simulink model "M4B11_modified_AGC_PI"  (R2025a)
settings: Solver=VariableStepAuto  StartTime=0.0  StopTime=100  RelTol=1e-3
InitFcn:
  | clear;
  | load('parameterinit.mat');
  | set_param('M4B11_modified_AGC_PI/Python2Sim','value','[0 0 0 0 0 0 0 0]');
  | acom=100;
  | bcom=50;
  | lam=100;
values from neighbouring files (symbols this model uses):
  ACgirdinit =     [datainit.mat]    (also in parameterinit.mat)
  AVm0 = [11.3576294988 11.3576294988]    [datainit.mat]    (also in parameterinit.mat)
  commun = [1 1 1 0]    [datainit.mat]    (also in initAll.m = [1,1,1,0]; parameterinit.mat)
  DataDelay = [0  0; 0  0; 0  0; 0  0]    [datainit.mat]    (also in initAll.m = 0.0*DataDelay; parameterinit.mat)
  ESinit =     [datainit.mat]    (also in parameterinit.mat)
  fB = 50    [datainit.mat]    (also in initAll.m; parameterinit.mat)
  Geninit =     [datainit.mat]    (also in initAll.m = Generator_init(opdata,SynMach_in_gidx); parameterinit.mat)
  SgridB = 100    [datainit.mat]    (also in initAll.m = resultsac.baseMVA; parameterinit.mat)
  wB = 314.159265359    [datainit.mat]    (also in initAll.m; parameterinit.mat)
  Windinit =     [datainit.mat]    (also in parameterinit.mat)
undefined symbols (not defined in the file or in its folder): c1, c2, c3, c4, c5, c6, cp_nom, lambda_nom, P_wind_base, Pelec_base, Pnom
libraries: spsBistableLib x9, slpidlib x2, simulink_extras x2
(part 3 of 6)

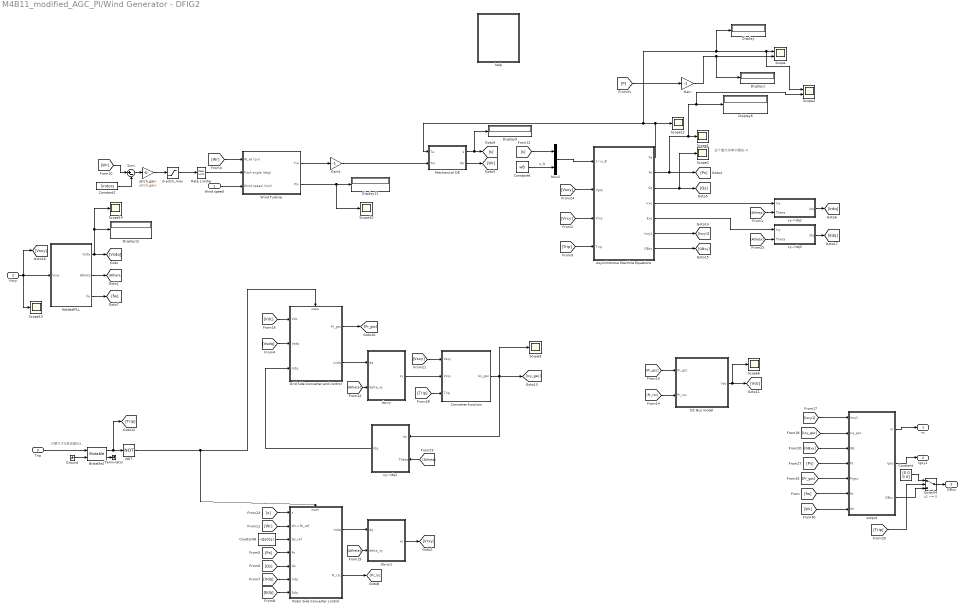
== system M4B11_modified_AGC_PI/Wind Generator - DFIG2 ==
  note: 只要大于0就会输出1
  note: 这个最大功率大概在-4
  Wind speed : Inport
  Vsxy : Inport  Port=2
  Trip : Inport  Port=3
  0-pitch_max : Saturate  UpperLimit=pitch_max  LowerLimit=0
  "Asynchronous Machine Equations " : Subsystem
  Bistable2 : spsBistableLib/Bistable  Qpriority=Set  ic=0  Ts=0
  Constant : Constant  Value=[0 0 0 0]
  Constant2 : Constant  Value=Srotors
  Constant6 : Constant  Value=wB
  Constant8 : Constant  Value=-Qs0(1)
  Converter function : Subsystem
  DC Bus model : Subsystem
  Display{,1,6,9,11..12} (6 alike) : Display
  Gain : Gain  Gain=-1
  Gain1 : Gain  Gain=-1
  Grid Side Converter and control : Subsystem
  Ground : Ground
  Mechanical DE : Subsystem
  Mux2 : Mux  Inputs=2
  NOT : Logic  Operator=NOT  AllPortsSameDT=off  OutDataTypeStr=boolean
  NoIdealPLL : Subsystem  VariantControl=Noideal_PLL_Wind1
  "Rate Limiter   " : RateLimiter  RisingSlewLimit=pitch_rate  FallingSlewLimit=-pitch_rate
  Rotor Side Converter control : Subsystem
  Scope : Scope  NumInputPorts=2
      settings: ActiveDisplayYMinimum=-1.1471  ActiveDisplayYMaximum=-0.81376
  Scope{1..3,6,10,12..14} (8 alike) : Scope
      Scope1 settings: ActiveDisplayYMinimum=-2.187000000000014  ActiveDisplayYMaximum=-2.186999999999987  DataLoggingVariableName=ScopeData2
      Scope10 settings: ActiveDisplayYMinimum=0.84538  ActiveDisplayYMaximum=0.84729
      Scope12 settings: ActiveDisplayYMinimum=-1.99497  ActiveDisplayYMaximum=-0.90484  DataLoggingVariableName=ScopeData6
      Scope13 settings: ActiveDisplayYMinimum=-1.25875  ActiveDisplayYMaximum=1.25908  DataLoggingVariableName=ScopeData2
      Scope14 settings: ActiveDisplayYMinimum=1.003489  ActiveDisplayYMaximum=1.0035  DataLoggingVariableName=ScopeData3
      Scope2 settings: ActiveDisplayYMinimum=-0.00085  ActiveDisplayYMaximum=0.00099  DataLoggingVariableName=ScopeData2
      Scope3 settings: ActiveDisplayYMinimum=-0.01172  ActiveDisplayYMaximum=0.10551
      Scope6 settings: ActiveDisplayYMinimum=2.82799999999992  ActiveDisplayYMaximum=2.82800000000004  DataLoggingVariableName=ScopeData5
  Scope4 : Scope  NumInputPorts=2
      settings: ActiveDisplayYMinimum=-1.13533  ActiveDisplayYMaximum=-0.91965  DataLoggingVariableName=ScopeData2
  Sum : Sum  Inputs=|+-  SaturateOnIntegerOverflow=on
  Switch4 : Switch  Criteria=u2 ~= 0  Threshold=0.5  InputSameDT=off
  Terminator : Terminator
  Wind Turbine : Subsystem
  dq-xy : Subsystem
  dq-xy1 : Subsystem
  help : Subsystem
  output : Subsystem
  pitch_gain : Gain  Gain=pitch_gain  SaturateOnIntegerOverflow=on  OutDataTypeStr=Inherit: Same as input  ParamDataTypeStr=Inherit: Same as input
  xy->dq1 : Subsystem
  xy->dq2 : Subsystem
  xy->dq3 : Subsystem
  m : Outport
  Igxy1 : Outport  Port=2
  GBxy : Outport  Port=3
  wires:
  [Wr] -> output/7(Wr)
  Gain1/1 -> Mechanical DE/2(Tm)
  output/3(GBxy) -> Switch4/3
  Switch4/1 -> GBxy/1
  Constant/1 -> Switch4/1
  [Trip] -> Switch4/2
  [Trip] -> Converter function/3(Trip)
  [Trip] -> "Asynchronous Machine Equations "/4("Trip ")
  [Wr] -> Sum/1
  0-pitch_max/1 -> "Rate Limiter   "/1
  pitch_gain/1 -> 0-pitch_max/1
  Constant2/1 -> Sum/2
  Sum/1 -> pitch_gain/1
  NOT/1 -> Rotor Side Converter control/Enable, Grid Side Converter and control/Enable
  Trip/1 -> Bistable2/1
  Bistable2/2 -> Terminator/1
  Bistable2/1 -> NOT/1, [Trip]
  Ground/1 -> Bistable2/2
  [fw] -> output/6(fw)
  [Pr_gsc] -> output/5(Prgsc)
  [Ps] -> output/4(Ps)
  output/1(m) -> m/1
  [Isxy1] -> output/1(Isxy1)
  [Ixy_gsc] -> output/2(Ixy_gsc)
  output/2(Igxy) -> Igxy1/1
  xy->dq3/1(Idq) -> [Edq]
  [Atheta] -> xy->dq3/2(Theta)
  xy->dq2/1(Idq) -> [Irdq]
  [Atheta] -> xy->dq2/2(Theta)
  dq-xy1/1(xy) -> [Vrxy]
  [Atheta] -> dq-xy1/2(delta_xy)
  xy->dq1/1(Idq) -> Grid Side Converter and control/3(Icdq)
  [Atheta] -> xy->dq1/2(Theta)
  [Atheta] -> dq-xy/2(delta_xy)
  dq-xy/1(xy) -> Converter function/2(Vcxy)
  Grid Side Converter and control/2(ucdq) -> dq-xy/1(dq)
  [Vsxy] -> Converter function/1(Vsxy)
  NoIdealPLL/3(fw) -> [fw]
  Vsxy/1 -> [Vsxy], Scope13/1, NoIdealPLL/1(Vsxy)
  [GBxy] -> output/3(GB)
  [Pr_rsc] -> DC Bus model/2(Pr_rsc)
  "Asynchronous Machine Equations "/1(Te) -> Scope12/1, Display/1, Scope4/1, Scope/1, Mechanical DE/1(Te)
  Constant8/1 -> Rotor Side Converter control/3(Qs_ref)
  [Wr] -> Wind Turbine/1(W_wt (pu))
  "Asynchronous Machine Equations "/4(Irxy) -> xy->dq2/1(Ixy)
  Converter function/1(Ixy_gsc) -> [Ixy_gsc], xy->dq1/1(Ixy), Scope3/1
  [Vrxy] -> "Asynchronous Machine Equations "/3(Vrxy)
  "Asynchronous Machine Equations "/6(Isxy1) -> [Isxy1]
  [Qs] -> Rotor Side Converter control/5(Qs)
  [Vdc] -> Grid Side Converter and control/1(Vdc)
  [Pr_gsc] -> DC Bus model/1(Pr_gsc)
  "Asynchronous Machine Equations "/2(Ps) -> Scope1/1, Scope4/2, Display6/1, [Ps]
  Mechanical DE/1("s ") -> [s], Display9/1
  [s] -> Mux2/1
  [Vsdq] -> Grid Side Converter and control/2(Vsdq)
  Grid Side Converter and control/1(Pr_gsc) -> [Pr_gsc]
  NoIdealPLL/2(Atheta) -> [Atheta]
  DC Bus model/1(Vdc) -> [Vdc], Scope6/1
  [Vsxy] -> "Asynchronous Machine Equations "/2(Vgxy)
  Wind Turbine/1(Tm) -> Gain1/1
  [Irdq] -> Rotor Side Converter control/6(Irdq)
  Mux2/1 -> "Asynchronous Machine Equations "/1(s / ω_B)
  "Asynchronous Machine Equations "/7(GBxy) -> [GBxy]
  "Rate Limiter   "/1 -> Wind Turbine/2(Pitch angle (deg))
  NoIdealPLL/1(Vsdq) -> Display12/1, Scope14/1, [Vsdq]
  [s] -> Rotor Side Converter control/1(s)
  Rotor Side Converter control/2(Pr_rsc) -> [Pr_rsc]
  Mechanical DE/2(Wr) -> [Wr]
  [Wr] -> Rotor Side Converter control/2(Wr->Ps_ref)
  Wind Turbine/2(Pm) -> Display11/1, Scope10/1
  "Asynchronous Machine Equations "/3(Qs) -> [Qs], Scope2/1
  Wind speed/1 -> Wind Turbine/3(Wind speed (m/s))
  [Ps] -> Rotor Side Converter control/4(Ps)
  Rotor Side Converter control/1(Vrdq) -> dq-xy1/1(dq)
  [Edq] -> Rotor Side Converter control/7(Edq)
  Constant6/1 -> Mux2/2  "w_B"
  "Asynchronous Machine Equations "/5(Exy) -> xy->dq3/1(Ixy)
  [P] -> Gain/1
  Gain/1 -> Display1/1, Scope/2

== system M4B11_modified_AGC_PI/ES1/ control1 ==
  usdq : Inport
  isdq : Inport  Port=2
  delta : Inport  Port=3
  Enable : EnablePort
  Add : Sum  Inputs=|-+
  Add2 : Sum  Inputs=|-+
  Add3 : Sum
  Add4 : Sum  Inputs=-+
  Add6 : Sum  Inputs=|++
  Add7 : Sum  Inputs=+-
  Complex to Magnitude-Angle : ComplexToMagnitudeAngle
  Complex to Real-Imag1 : ComplexToRealImag
  Constant : Constant
  Constant1 : Constant  Value=usd0
  Constant2 : Constant  Value=0
  Constant3 : Constant  Value=Q0
  Constant4 : Constant
  Demux : Demux  Outputs=2
  Demux1 : Demux  Outputs=2
  Gain : Gain  Gain=0.01
  Gain1 : Gain  Gain=-1
  K5 : Gain  Gain=Lpr  SaturateOnIntegerOverflow=on  OutDataTypeStr=Inherit: Same as input  ParamDataTypeStr=Inherit: Same as input
  K6 : Gain  Gain=Lpr  SaturateOnIntegerOverflow=on  OutDataTypeStr=Inherit: Same as input  ParamDataTypeStr=Inherit: Same as input
  Magnitude-Angle to Complex : MagnitudeAngleToComplex
  Product{1,4..6} (4 alike) : Product  RndMeth=Zero
  Real-Imag to Complex : RealImagToComplex
  Scope : Scope
      settings: ActiveDisplayYMinimum=-1.90229  ActiveDisplayYMaximum=-1.00495  DataLoggingVariableName=ScopeData6
  Scope1 : Scope
      settings: ActiveDisplayYMinimum=1.01143  ActiveDisplayYMaximum=1.18506  DataLoggingVariableName=ScopeData8
  Scope2 : Scope  NumInputPorts=2
      settings: ActiveDisplayYMinimum=-1E-15  ActiveDisplayYMaximum=1.3E-14  DataLoggingVariableName=ScopeData9
  Scope3 : Scope  NumInputPorts=2
      settings: ActiveDisplayYMinimum=-0.06902  ActiveDisplayYMaximum=1.69489  DataLoggingVariableName=ScopeData4
  Scope7 : Scope  NumInputPorts=2
      settings: ActiveDisplayYMinimum=-1.01296  ActiveDisplayYMaximum=-0.62415
  Sum : Sum  Inputs=|+-
  Sum2 : Sum  Inputs=|+-  SaturateOnIntegerOverflow=on
  Sum23 : Sum  Inputs=|+-  SaturateOnIntegerOverflow=on
  Sum9 : Sum  Inputs=|+-  SaturateOnIntegerOverflow=on
  control_AC_voltage : Subsystem  VariantControl=VSC1q_Variant2
  control_AC_voltage1 : Subsystem  VariantControl=VSC1q_Variant2
  in_D_PI : Subsystem  mask{KP_=KpId_VSC_A, KI_=KiId_VSC_A, Upper_limit=inf, Lower_limit=-inf, Upper_saturation_limit=inf, Lower_saturation_limit=-inf, integrator_init=Md_A_0}
      mask prompts: KP_ "比例系数P"; KI_ "积分系数I"; Upper_limit "限幅上限"; Lower_limit "限幅下限"; Upper_saturation_limit "积分饱和上限"; Lower_saturation_limit "积分饱和下限"; integrator_init "积分初始值"
      mask DialogControl Container4 Prompt: 控制参数
      mask DialogControl Container5 Prompt: 初始值
      mask Display: disp('PI')
  in_Q_PI : Subsystem  mask{KP_=KpIq_VSC_A, KI_=KiIq_VSC_A, Upper_limit=inf, Lower_limit=-inf, Upper_saturation_limit=inf, Lower_saturation_limit=-inf, integrator_init=Mq_A_0}
      mask prompts: KP_ "比例系数P"; KI_ "积分系数I"; Upper_limit "限幅上限"; Lower_limit "限幅下限"; Upper_saturation_limit "积分饱和上限"; Lower_saturation_limit "积分饱和下限"; integrator_init "积分初始值"
      mask DialogControl Container4 Prompt: 控制参数
      mask DialogControl Container5 Prompt: 初始值
      mask Display: disp('PI')
  ucx : Outport
  ucy : Outport  Port=2
  wires:
  Magnitude-Angle to Complex/1 -> Complex to Real-Imag1/1
  Add/1 -> Real-Imag to Complex/2
  Add2/1 -> Real-Imag to Complex/1
  delta/1 -> Add6/2
  Add6/1 -> Magnitude-Angle to Complex/2
  Complex to Magnitude-Angle/2 -> Add6/1
  Sum9/1 -> in_D_PI/1(In1)
  K5/1 -> Add3/1
  [usd] -> Add3/2
  Add3/1 -> Add2/2
  in_D_PI/1(Out1) -> Add2/1
  Constant/1 -> Product4/2
  [isq] -> Product4/1
  [isd] -> Scope7/2, Sum9/2
  Product4/1 -> K5/1
  Demux1/1 -> [isd]
  Demux/1 -> [usd]
  Demux1/2 -> [isq]
  Demux/2 -> [usq]
  isdq/1 -> Demux1/1
  usdq/1 -> Demux/1
  [usq] -> Add4/2
  K6/1 -> Add4/1
  in_Q_PI/1(Out1) -> Add/1
  Sum23/1 -> in_Q_PI/1(In1)
  [isd] -> Product1/1
  [isq] -> Sum23/2, Scope3/2
  Product1/1 -> K6/1
  Constant4/1 -> Product1/2
  Add4/1 -> Add/2
  Real-Imag to Complex/1 -> Complex to Magnitude-Angle/1
  Complex to Magnitude-Angle/1 -> Magnitude-Angle to Complex/1
  Complex to Real-Imag1/1 -> ucx/1
  Complex to Real-Imag1/2 -> ucy/1
  [usd] -> Scope1/1, control_AC_voltage/1(usd)
  control_AC_voltage/1(isdref) -> Scope7/1, Sum9/1
  [isq] -> Product5/2
  Product5/1 -> Add7/2
  [usd] -> Product5/1
  [isd] -> Product6/2
  Product6/1 -> Add7/1
  [usq] -> Product6/1
  Gain/1 -> Sum/2
  control_AC_voltage1/1(isqref) -> Scope3/1, Sum23/1
  [usq] -> Scope2/1, control_AC_voltage1/1(usq)
  Constant2/1 -> Scope2/2, control_AC_voltage1/2(usqref)
  Add7/1 -> Scope/1, Gain1/1
  Sum2/1 -> Gain/1
  Constant3/1 -> Sum2/2
  Gain1/1 -> Sum2/1
  Sum/1 -> control_AC_voltage/2(usdref)
  Constant1/1 -> Sum/1

== system M4B11_modified_AGC_PI/ES1/in_D_PI ==
  In1 : Inport
  Ki : Gain  Gain=KI_  SaturateOnIntegerOverflow=on  OutDataTypeStr=Inherit: Same as input  ParamDataTypeStr=Inherit: Same as input
  Kp : Gain  Gain=KP_  SaturateOnIntegerOverflow=on  OutDataTypeStr=Inherit: Same as input  ParamDataTypeStr=Inherit: Same as input
  Saturation2 : Saturate  UpperLimit=Upper_limit  LowerLimit=Lower_limit
  Sum12 : Sum  SaturateOnIntegerOverflow=on
  integrator : Integrator  InitialCondition=integrator_init  LimitOutput=on  UpperSaturationLimit=Upper_saturation_limit  LowerSaturationLimit=Lower_saturation_limit
  Out1 : Outport
  wires:
  In1/1 -> Ki/1, Kp/1
  Kp/1 -> Sum12/2
  Ki/1 -> integrator/1
  integrator/1 -> Sum12/1
  Saturation2/1 -> Out1/1
  Sum12/1 -> Saturation2/1

== system M4B11_modified_AGC_PI/ES1/output ==
  is_xy : Inport
  Pe : Inport  Port=2
  Brecx : Constant  Value=0
  Brecy : Constant  Value=0
  Bus Creator : BusCreator  Inputs=4
  Constant : Constant
  Gain : Gain  Gain=SvscB./SgridB
  Gain1 : Gain  Gain=-1
  Gain2 : Gain  Gain=-1
  Gain6 : Gain
  Grecx : Constant  Value=0
  Grecy : Constant  Value=0
  Mux3 : Mux
  Sum : Sum  Inputs=|++
  m : Outport
  isxy : Outport  Port=2
  GBxy : Outport  Port=3
  wires:
  Bus Creator/1 -> m/1
  Gain6/1 -> GBxy/1, Bus Creator/4  "GBxy"
  Mux3/1 -> Gain6/1
  Grecx/1 -> Mux3/1
  Brecx/1 -> Mux3/3
  Grecy/1 -> Mux3/2
  Brecy/1 -> Mux3/4
  Gain1/1 -> isxy/1, Bus Creator/1  "is_xy"
  Gain2/1 -> Bus Creator/2  "Pe"
  Gain/1 -> Gain1/1  "is_xy"
  Pe/1 -> Gain2/1  "Pe"
  [WreES1] -> Sum/1  "Pe"
  Constant/1 -> Sum/2
  Sum/1 -> Bus Creator/3  "w"
  is_xy/1 -> Gain/1

== system M4B11_modified_AGC_PI/ES1/xy->dq ==
  Ixy : Inport
  Theta : Inport  Port=2
  Complex to Magnitude-Angle : ComplexToMagnitudeAngle
  Complex to Real-Imag : ComplexToRealImag
  Demux1 : Demux  Outputs=2
      settings: DisplayOption=none
  Magnitude-Angle to Complex : MagnitudeAngleToComplex
  Mux : Mux  Inputs=2
  Real-Imag to Complex : RealImagToComplex
  Scope : Scope
      settings: ActiveDisplayYMinimum=3.11918  ActiveDisplayYMaximum=3.16079
  Scope1 : Scope
      settings: ActiveDisplayYMinimum=2.59405  ActiveDisplayYMaximum=3.13201  DataLoggingVariableName=ScopeData3
  Sum1 : Sum  Inputs=|+-  SaturateOnIntegerOverflow=on
  Idq : Outport
  wires:
  Complex to Magnitude-Angle/1 -> Magnitude-Angle to Complex/1
  Theta/1 -> Sum1/2
  Complex to Magnitude-Angle/2 -> Sum1/1, Scope1/1
  Demux1/1 -> Real-Imag to Complex/1
  Complex to Real-Imag/2 -> Mux/2  "Iq"
  Mux/1 -> Idq/1
  Complex to Real-Imag/1 -> Mux/1  "Id"
  Magnitude-Angle to Complex/1 -> Complex to Real-Imag/1
  Sum1/1 -> Magnitude-Angle to Complex/2, Scope/1
  Demux1/2 -> Real-Imag to Complex/2
  Real-Imag to Complex/1 -> Complex to Magnitude-Angle/1
  Ixy/1 -> Demux1/1

== system M4B11_modified_AGC_PI/ES2/ control1 ==
  usdq : Inport
  isdq : Inport  Port=2
  delta : Inport  Port=3
  Enable : EnablePort
  Add : Sum  Inputs=|-+
  Add2 : Sum  Inputs=|-+
  Add3 : Sum
  Add4 : Sum  Inputs=-+
  Add6 : Sum  Inputs=|++
  Add7 : Sum  Inputs=+-
  Complex to Magnitude-Angle : ComplexToMagnitudeAngle
  Complex to Real-Imag1 : ComplexToRealImag
  Constant : Constant
  Constant1 : Constant  Value=usd0
  Constant2 : Constant  Value=0
  Constant3 : Constant  Value=Q0
  Constant4 : Constant
  Demux : Demux  Outputs=2
  Demux1 : Demux  Outputs=2
  Gain : Gain  Gain=0.01
  Gain1 : Gain  Gain=-1
  K5 : Gain  Gain=Lpr  SaturateOnIntegerOverflow=on  OutDataTypeStr=Inherit: Same as input  ParamDataTypeStr=Inherit: Same as input
  K6 : Gain  Gain=Lpr  SaturateOnIntegerOverflow=on  OutDataTypeStr=Inherit: Same as input  ParamDataTypeStr=Inherit: Same as input
  Magnitude-Angle to Complex : MagnitudeAngleToComplex
  Product{1,4..6} (4 alike) : Product  RndMeth=Zero
  Real-Imag to Complex : RealImagToComplex
  Scope{,1..2,7} (4 alike) : Scope
      Scope settings: ActiveDisplayYMinimum=-2.62202  ActiveDisplayYMaximum=-0.62202  DataLoggingVariableName=ScopeData6
      Scope1 settings: ActiveDisplayYMinimum=0.03  ActiveDisplayYMaximum=2.03  DataLoggingVariableName=ScopeData8
      Scope2 settings: ActiveDisplayYMinimum=-1.2875  ActiveDisplayYMaximum=1.2875  DataLoggingVariableName=ScopeData9
      Scope7 settings: ActiveDisplayYMinimum=-7.47817  ActiveDisplayYMaximum=-5.47817
  Sum : Sum  Inputs=|+-
  Sum2 : Sum  Inputs=|+-  SaturateOnIntegerOverflow=on
  Sum23 : Sum  Inputs=|+-  SaturateOnIntegerOverflow=on
  Sum9 : Sum  Inputs=|+-  SaturateOnIntegerOverflow=on
  control_AC_voltage : Subsystem  VariantControl=VSC1q_Variant2
  control_AC_voltage1 : Subsystem  VariantControl=VSC1q_Variant2
  in_D_PI : Subsystem  mask{KP_=KpId_VSC_A, KI_=KiId_VSC_A, Upper_limit=inf, Lower_limit=-inf, Upper_saturation_limit=inf, Lower_saturation_limit=-inf, integrator_init=Md_A_0}
      mask prompts: KP_ "比例系数P"; KI_ "积分系数I"; Upper_limit "限幅上限"; Lower_limit "限幅下限"; Upper_saturation_limit "积分饱和上限"; Lower_saturation_limit "积分饱和下限"; integrator_init "积分初始值"
      mask DialogControl Container4 Prompt: 控制参数
      mask DialogControl Container5 Prompt: 初始值
      mask Display: disp('PI')
  in_Q_PI : Subsystem  mask{KP_=KpIq_VSC_A, KI_=KiIq_VSC_A, Upper_limit=inf, Lower_limit=-inf, Upper_saturation_limit=inf, Lower_saturation_limit=-inf, integrator_init=Mq_A_0}
      mask prompts: KP_ "比例系数P"; KI_ "积分系数I"; Upper_limit "限幅上限"; Lower_limit "限幅下限"; Upper_saturation_limit "积分饱和上限"; Lower_saturation_limit "积分饱和下限"; integrator_init "积分初始值"
      mask DialogControl Container4 Prompt: 控制参数
      mask DialogControl Container5 Prompt: 初始值
      mask Display: disp('PI')
  ucx : Outport
  ucy : Outport  Port=2
  wires:
  Magnitude-Angle to Complex/1 -> Complex to Real-Imag1/1
  Add/1 -> Real-Imag to Complex/2
  Add2/1 -> Real-Imag to Complex/1
  delta/1 -> Add6/2
  Add6/1 -> Magnitude-Angle to Complex/2
  Complex to Magnitude-Angle/2 -> Add6/1
  Sum9/1 -> in_D_PI/1(In1)
  K5/1 -> Add3/1
  [usd] -> Add3/2
  Add3/1 -> Add2/2
  in_D_PI/1(Out1) -> Add2/1
  Constant/1 -> Product4/2
  [isq] -> Product4/1
  [isd] -> Sum9/2
  Product4/1 -> K5/1
  Demux1/1 -> [isd]
  Demux/1 -> [usd]
  Demux1/2 -> [isq]
  Demux/2 -> [usq]
  isdq/1 -> Demux1/1
  usdq/1 -> Demux/1
  [usq] -> Add4/2
  K6/1 -> Add4/1
  in_Q_PI/1(Out1) -> Add/1
  Sum23/1 -> in_Q_PI/1(In1)
  [isd] -> Product1/1
  [isq] -> Sum23/2
  Product1/1 -> K6/1
  Constant4/1 -> Product1/2
  Add4/1 -> Add/2
  Real-Imag to Complex/1 -> Complex to Magnitude-Angle/1
  Complex to Magnitude-Angle/1 -> Magnitude-Angle to Complex/1
  Complex to Real-Imag1/1 -> ucx/1
  Complex to Real-Imag1/2 -> ucy/1
  [usd] -> Scope1/1, control_AC_voltage/1(usd)
  control_AC_voltage/1(isdref) -> Scope7/1, Sum9/1
  [isq] -> Product5/2
  Product5/1 -> Add7/2
  [usd] -> Product5/1
  [isd] -> Product6/2
  Product6/1 -> Add7/1
  [usq] -> Product6/1
  Gain/1 -> Sum/2
  control_AC_voltage1/1(isqref) -> Sum23/1
  [usq] -> Scope2/1, control_AC_voltage1/1(usq)
  Constant2/1 -> control_AC_voltage1/2(usqref)
  Add7/1 -> Scope/1, Gain1/1
  Sum2/1 -> Gain/1
  Constant3/1 -> Sum2/2
  Gain1/1 -> Sum2/1
  Sum/1 -> control_AC_voltage/2(usdref)
  Constant1/1 -> Sum/1

== system M4B11_modified_AGC_PI/ES2/output ==
  is_xy : Inport
  Pe : Inport  Port=2
  Brecx : Constant  Value=0
  Brecy : Constant  Value=0
  Bus Creator : BusCreator  Inputs=4
  Constant : Constant
  Gain : Gain  Gain=SvscB./SgridB
  Gain1 : Gain  Gain=-1
  Gain2 : Gain  Gain=-1
  Gain6 : Gain
  Grecx : Constant  Value=0
  Grecy : Constant  Value=0
  Mux3 : Mux
  Sum : Sum  Inputs=|++
  m : Outport
  isxy : Outport  Port=2
  GBxy : Outport  Port=3
  wires:
  Bus Creator/1 -> m/1
  Gain6/1 -> GBxy/1, Bus Creator/4  "GBxy"
  Mux3/1 -> Gain6/1
  Grecx/1 -> Mux3/1
  Brecx/1 -> Mux3/3
  Grecy/1 -> Mux3/2
  Brecy/1 -> Mux3/4
  Gain1/1 -> isxy/1, Bus Creator/1  "is_xy"
  Gain2/1 -> Bus Creator/2  "Pe"
  Gain/1 -> Gain1/1  "is_xy"
  Pe/1 -> Gain2/1  "Pe"
  Constant/1 -> Sum/2
  [WreES2] -> Sum/1  "Pe"
  Sum/1 -> Bus Creator/3  "w"
  is_xy/1 -> Gain/1

== system M4B11_modified_AGC_PI/ES2/xy->dq ==
  Ixy : Inport
  Theta : Inport  Port=2
  Complex to Magnitude-Angle : ComplexToMagnitudeAngle
  Complex to Real-Imag : ComplexToRealImag
  Demux1 : Demux  Outputs=2
      settings: DisplayOption=none
  Magnitude-Angle to Complex : MagnitudeAngleToComplex
  Mux : Mux  Inputs=2
  Real-Imag to Complex : RealImagToComplex
  Scope : Scope
      settings: ActiveDisplayYMinimum=3.11918  ActiveDisplayYMaximum=3.16079
  Scope1 : Scope
      settings: ActiveDisplayYMinimum=2.59405  ActiveDisplayYMaximum=3.13201  DataLoggingVariableName=ScopeData3
  Sum1 : Sum  Inputs=|+-  SaturateOnIntegerOverflow=on
  Idq : Outport
  wires:
  Complex to Magnitude-Angle/1 -> Magnitude-Angle to Complex/1
  Theta/1 -> Sum1/2
  Complex to Magnitude-Angle/2 -> Sum1/1, Scope1/1
  Demux1/1 -> Real-Imag to Complex/1
  Complex to Real-Imag/2 -> Mux/2  "Iq"
  Mux/1 -> Idq/1
  Complex to Real-Imag/1 -> Mux/1  "Id"
  Magnitude-Angle to Complex/1 -> Complex to Real-Imag/1
  Sum1/1 -> Magnitude-Angle to Complex/2, Scope/1
  Demux1/2 -> Real-Imag to Complex/2
  Real-Imag to Complex/1 -> Complex to Magnitude-Angle/1
  Ixy/1 -> Demux1/1

== system M4B11_modified_AGC_PI/ES3/ control1 ==
  usdq : Inport
  isdq : Inport  Port=2
  delta : Inport  Port=3
  Enable : EnablePort
  Add : Sum  Inputs=|-+
  Add2 : Sum  Inputs=|-+
  Add3 : Sum
  Add4 : Sum  Inputs=-+
  Add6 : Sum  Inputs=|++
  Add7 : Sum  Inputs=+-
  Complex to Magnitude-Angle : ComplexToMagnitudeAngle
  Complex to Real-Imag1 : ComplexToRealImag
  Constant : Constant
  Constant1 : Constant  Value=usd0
  Constant2 : Constant  Value=0
  Constant3 : Constant  Value=Q0
  Constant4 : Constant
  Demux : Demux  Outputs=2
  Demux1 : Demux  Outputs=2
  Gain : Gain  Gain=0.01
  Gain1 : Gain  Gain=-1
  K5 : Gain  Gain=Lpr  SaturateOnIntegerOverflow=on  OutDataTypeStr=Inherit: Same as input  ParamDataTypeStr=Inherit: Same as input
  K6 : Gain  Gain=Lpr  SaturateOnIntegerOverflow=on  OutDataTypeStr=Inherit: Same as input  ParamDataTypeStr=Inherit: Same as input
  Magnitude-Angle to Complex : MagnitudeAngleToComplex
  Product{1,4..6} (4 alike) : Product  RndMeth=Zero
  Real-Imag to Complex : RealImagToComplex
  Scope{,1..2,7} (4 alike) : Scope
      Scope settings: ActiveDisplayYMinimum=-2.62202  ActiveDisplayYMaximum=-0.62202  DataLoggingVariableName=ScopeData6
      Scope1 settings: ActiveDisplayYMinimum=0.03  ActiveDisplayYMaximum=2.03  DataLoggingVariableName=ScopeData8
      Scope2 settings: ActiveDisplayYMinimum=-1.2875  ActiveDisplayYMaximum=1.2875  DataLoggingVariableName=ScopeData9
      Scope7 settings: ActiveDisplayYMinimum=-7.47817  ActiveDisplayYMaximum=-5.47817
  Sum : Sum  Inputs=|+-
  Sum2 : Sum  Inputs=|+-  SaturateOnIntegerOverflow=on
  Sum23 : Sum  Inputs=|+-  SaturateOnIntegerOverflow=on
  Sum9 : Sum  Inputs=|+-  SaturateOnIntegerOverflow=on
  control_AC_voltage : Subsystem  VariantControl=VSC1q_Variant2
  control_AC_voltage1 : Subsystem  VariantControl=VSC1q_Variant2
  in_D_PI : Subsystem  mask{KP_=KpId_VSC_A, KI_=KiId_VSC_A, Upper_limit=inf, Lower_limit=-inf, Upper_saturation_limit=inf, Lower_saturation_limit=-inf, integrator_init=Md_A_0}
      mask prompts: KP_ "比例系数P"; KI_ "积分系数I"; Upper_limit "限幅上限"; Lower_limit "限幅下限"; Upper_saturation_limit "积分饱和上限"; Lower_saturation_limit "积分饱和下限"; integrator_init "积分初始值"
      mask DialogControl Container4 Prompt: 控制参数
      mask DialogControl Container5 Prompt: 初始值
      mask Display: disp('PI')
  in_Q_PI : Subsystem  mask{KP_=KpIq_VSC_A, KI_=KiIq_VSC_A, Upper_limit=inf, Lower_limit=-inf, Upper_saturation_limit=inf, Lower_saturation_limit=-inf, integrator_init=Mq_A_0}
      mask prompts: KP_ "比例系数P"; KI_ "积分系数I"; Upper_limit "限幅上限"; Lower_limit "限幅下限"; Upper_saturation_limit "积分饱和上限"; Lower_saturation_limit "积分饱和下限"; integrator_init "积分初始值"
      mask DialogControl Container4 Prompt: 控制参数
      mask DialogControl Container5 Prompt: 初始值
      mask Display: disp('PI')
  ucx : Outport
  ucy : Outport  Port=2
  wires:
  Magnitude-Angle to Complex/1 -> Complex to Real-Imag1/1
  Add/1 -> Real-Imag to Complex/2
  Add2/1 -> Real-Imag to Complex/1
  delta/1 -> Add6/2
  Add6/1 -> Magnitude-Angle to Complex/2
  Complex to Magnitude-Angle/2 -> Add6/1
  Sum9/1 -> in_D_PI/1(In1)
  K5/1 -> Add3/1
  [usd] -> Add3/2
  Add3/1 -> Add2/2
  in_D_PI/1(Out1) -> Add2/1
  Constant/1 -> Product4/2
  [isq] -> Product4/1
  [isd] -> Sum9/2
  Product4/1 -> K5/1
  Demux1/1 -> [isd]
  Demux/1 -> [usd]
  Demux1/2 -> [isq]
  Demux/2 -> [usq]
  isdq/1 -> Demux1/1
  usdq/1 -> Demux/1
  [usq] -> Add4/2
  K6/1 -> Add4/1
  in_Q_PI/1(Out1) -> Add/1
  Sum23/1 -> in_Q_PI/1(In1)
  [isd] -> Product1/1
  [isq] -> Sum23/2
  Product1/1 -> K6/1
  Constant4/1 -> Product1/2
  Add4/1 -> Add/2
  Real-Imag to Complex/1 -> Complex to Magnitude-Angle/1
  Complex to Magnitude-Angle/1 -> Magnitude-Angle to Complex/1
  Complex to Real-Imag1/1 -> ucx/1
  Complex to Real-Imag1/2 -> ucy/1
  [usd] -> Scope1/1, control_AC_voltage/1(usd)
  control_AC_voltage/1(isdref) -> Scope7/1, Sum9/1
  [isq] -> Product5/2
  Product5/1 -> Add7/2
  [usd] -> Product5/1
  [isd] -> Product6/2
  Product6/1 -> Add7/1
  [usq] -> Product6/1
  Gain/1 -> Sum/2
  control_AC_voltage1/1(isqref) -> Sum23/1
  [usq] -> Scope2/1, control_AC_voltage1/1(usq)
  Constant2/1 -> control_AC_voltage1/2(usqref)
  Add7/1 -> Scope/1, Gain1/1
  Sum2/1 -> Gain/1
  Constant3/1 -> Sum2/2
  Gain1/1 -> Sum2/1
  Sum/1 -> control_AC_voltage/2(usdref)
  Constant1/1 -> Sum/1

== system M4B11_modified_AGC_PI/ES3/in_D_PI ==
  In1 : Inport
  Ki : Gain  Gain=KI_  SaturateOnIntegerOverflow=on  OutDataTypeStr=Inherit: Same as input  ParamDataTypeStr=Inherit: Same as input
  Kp : Gain  Gain=KP_  SaturateOnIntegerOverflow=on  OutDataTypeStr=Inherit: Same as input  ParamDataTypeStr=Inherit: Same as input
  Saturation2 : Saturate  UpperLimit=Upper_limit  LowerLimit=Lower_limit
  Sum12 : Sum  SaturateOnIntegerOverflow=on
  integrator : Integrator  InitialCondition=integrator_init  LimitOutput=on  UpperSaturationLimit=Upper_saturation_limit  LowerSaturationLimit=Lower_saturation_limit
  Out1 : Outport
  wires:
  In1/1 -> Ki/1, Kp/1
  Kp/1 -> Sum12/2
  Ki/1 -> integrator/1
  integrator/1 -> Sum12/1
  Saturation2/1 -> Out1/1
  Sum12/1 -> Saturation2/1

== system M4B11_modified_AGC_PI/ES3/output ==
  is_xy : Inport
  Pe : Inport  Port=2
  Brecx : Constant  Value=0
  Brecy : Constant  Value=0
  Bus Creator : BusCreator  Inputs=4
  Constant : Constant
  Gain : Gain  Gain=SvscB./SgridB
  Gain1 : Gain  Gain=-1
  Gain2 : Gain  Gain=-1
  Gain6 : Gain
  Grecx : Constant  Value=0
  Grecy : Constant  Value=0
  Mux3 : Mux
  Sum : Sum  Inputs=|++
  m : Outport
  isxy : Outport  Port=2
  GBxy : Outport  Port=3
  wires:
  Bus Creator/1 -> m/1
  Gain6/1 -> GBxy/1, Bus Creator/4  "GBxy"
  Mux3/1 -> Gain6/1
  Grecx/1 -> Mux3/1
  Brecx/1 -> Mux3/3
  Grecy/1 -> Mux3/2
  Brecy/1 -> Mux3/4
  Gain1/1 -> isxy/1, Bus Creator/1  "is_xy"
  Gain2/1 -> Bus Creator/2  "Pe"
  Gain/1 -> Gain1/1  "is_xy"
  Pe/1 -> Gain2/1  "Pe"
  Constant/1 -> Sum/2
  [WreES3] -> Sum/1  "Pe"
  Sum/1 -> Bus Creator/3  "w"
  is_xy/1 -> Gain/1

== system M4B11_modified_AGC_PI/ES3/xy->dq ==
  Ixy : Inport
  Theta : Inport  Port=2
  Complex to Magnitude-Angle : ComplexToMagnitudeAngle
  Complex to Real-Imag : ComplexToRealImag
  Demux1 : Demux  Outputs=2
      settings: DisplayOption=none
  Magnitude-Angle to Complex : MagnitudeAngleToComplex
  Mux : Mux  Inputs=2
  Real-Imag to Complex : RealImagToComplex
  Scope : Scope
      settings: ActiveDisplayYMinimum=3.11918  ActiveDisplayYMaximum=3.16079
  Scope1 : Scope
      settings: ActiveDisplayYMinimum=2.59405  ActiveDisplayYMaximum=3.13201  DataLoggingVariableName=ScopeData3
  Sum1 : Sum  Inputs=|+-  SaturateOnIntegerOverflow=on
  Idq : Outport
  wires:
  Complex to Magnitude-Angle/1 -> Magnitude-Angle to Complex/1
  Theta/1 -> Sum1/2
  Complex to Magnitude-Angle/2 -> Sum1/1, Scope1/1
  Demux1/1 -> Real-Imag to Complex/1
  Complex to Real-Imag/2 -> Mux/2  "Iq"
  Mux/1 -> Idq/1
  Complex to Real-Imag/1 -> Mux/1  "Id"
  Magnitude-Angle to Complex/1 -> Complex to Real-Imag/1
  Sum1/1 -> Magnitude-Angle to Complex/2, Scope/1
  Demux1/2 -> Real-Imag to Complex/2
  Real-Imag to Complex/1 -> Complex to Magnitude-Angle/1
  Ixy/1 -> Demux1/1

== system M4B11_modified_AGC_PI/ES4/ control1 ==
  usdq : Inport
  isdq : Inport  Port=2
  delta : Inport  Port=3
  Enable : EnablePort
  Add : Sum  Inputs=|-+
  Add2 : Sum  Inputs=|-+
  Add3 : Sum
  Add4 : Sum  Inputs=-+
  Add6 : Sum  Inputs=|++
  Add7 : Sum  Inputs=+-
  Complex to Magnitude-Angle : ComplexToMagnitudeAngle
  Complex to Real-Imag1 : ComplexToRealImag
  Constant : Constant
  Constant1 : Constant  Value=usd0
  Constant2 : Constant  Value=0
  Constant3 : Constant  Value=Q0
  Constant4 : Constant
  Demux : Demux  Outputs=2
  Demux1 : Demux  Outputs=2
  Gain1 : Gain  Gain=-1
  Gain2 : Gain  Gain=0.01
  K5 : Gain  Gain=Lpr  SaturateOnIntegerOverflow=on  OutDataTypeStr=Inherit: Same as input  ParamDataTypeStr=Inherit: Same as input
  K6 : Gain  Gain=Lpr  SaturateOnIntegerOverflow=on  OutDataTypeStr=Inherit: Same as input  ParamDataTypeStr=Inherit: Same as input
  Magnitude-Angle to Complex : MagnitudeAngleToComplex
  Product{1,4..6} (4 alike) : Product  RndMeth=Zero
  Real-Imag to Complex : RealImagToComplex
  Scope{,1..2,7} (4 alike) : Scope
      Scope settings: ActiveDisplayYMinimum=-2.62202  ActiveDisplayYMaximum=-0.62202  DataLoggingVariableName=ScopeData6
      Scope1 settings: ActiveDisplayYMinimum=0.03  ActiveDisplayYMaximum=2.03  DataLoggingVariableName=ScopeData8
      Scope2 settings: ActiveDisplayYMinimum=-1.2875  ActiveDisplayYMaximum=1.2875  DataLoggingVariableName=ScopeData9
      Scope7 settings: ActiveDisplayYMinimum=-7.47817  ActiveDisplayYMaximum=-5.47817
  Sum : Sum  Inputs=|+-
  Sum2 : Sum  Inputs=|+-  SaturateOnIntegerOverflow=on
  Sum23 : Sum  Inputs=|+-  SaturateOnIntegerOverflow=on
  Sum9 : Sum  Inputs=|+-  SaturateOnIntegerOverflow=on
  control_AC_voltage : Subsystem  VariantControl=VSC1q_Variant2
  control_AC_voltage1 : Subsystem  VariantControl=VSC1q_Variant2
  in_D_PI : Subsystem  mask{KP_=KpId_VSC_A, KI_=KiId_VSC_A, Upper_limit=inf, Lower_limit=-inf, Upper_saturation_limit=inf, Lower_saturation_limit=-inf, integrator_init=Md_A_0}
      mask prompts: KP_ "比例系数P"; KI_ "积分系数I"; Upper_limit "限幅上限"; Lower_limit "限幅下限"; Upper_saturation_limit "积分饱和上限"; Lower_saturation_limit "积分饱和下限"; integrator_init "积分初始值"
      mask DialogControl Container4 Prompt: 控制参数
      mask DialogControl Container5 Prompt: 初始值
      mask Display: disp('PI')
  in_Q_PI : Subsystem  mask{KP_=KpIq_VSC_A, KI_=KiIq_VSC_A, Upper_limit=inf, Lower_limit=-inf, Upper_saturation_limit=inf, Lower_saturation_limit=-inf, integrator_init=Mq_A_0}
      mask prompts: KP_ "比例系数P"; KI_ "积分系数I"; Upper_limit "限幅上限"; Lower_limit "限幅下限"; Upper_saturation_limit "积分饱和上限"; Lower_saturation_limit "积分饱和下限"; integrator_init "积分初始值"
      mask DialogControl Container4 Prompt: 控制参数
      mask DialogControl Container5 Prompt: 初始值
      mask Display: disp('PI')
  ucx : Outport
  ucy : Outport  Port=2
  wires:
  Magnitude-Angle to Complex/1 -> Complex to Real-Imag1/1
  Add/1 -> Real-Imag to Complex/2
  Add2/1 -> Real-Imag to Complex/1
  delta/1 -> Add6/2
  Add6/1 -> Magnitude-Angle to Complex/2
  Complex to Magnitude-Angle/2 -> Add6/1
  Sum9/1 -> in_D_PI/1(In1)
  K5/1 -> Add3/1
  [usd] -> Add3/2
  Add3/1 -> Add2/2
  in_D_PI/1(Out1) -> Add2/1
  Constant/1 -> Product4/2
  [isq] -> Product4/1
  [isd] -> Sum9/2
  Product4/1 -> K5/1
  Demux1/1 -> [isd]
  Demux/1 -> [usd]
  Demux1/2 -> [isq]
  Demux/2 -> [usq]
  isdq/1 -> Demux1/1
  usdq/1 -> Demux/1
  [usq] -> Add4/2
  K6/1 -> Add4/1
  in_Q_PI/1(Out1) -> Add/1
  Sum23/1 -> in_Q_PI/1(In1)
  [isd] -> Product1/1
  [isq] -> Sum23/2
  Product1/1 -> K6/1
  Constant4/1 -> Product1/2
  Add4/1 -> Add/2
  Real-Imag to Complex/1 -> Complex to Magnitude-Angle/1
  Complex to Magnitude-Angle/1 -> Magnitude-Angle to Complex/1
  Complex to Real-Imag1/1 -> ucx/1
  Complex to Real-Imag1/2 -> ucy/1
  [usd] -> Scope1/1, control_AC_voltage/1(usd)
  control_AC_voltage/1(isdref) -> Scope7/1, Sum9/1
  [isq] -> Product5/2
  Product5/1 -> Add7/2
  [usd] -> Product5/1
  [isd] -> Product6/2
  Product6/1 -> Add7/1
  [usq] -> Product6/1
  Gain2/1 -> Sum/2
  control_AC_voltage1/1(isqref) -> Sum23/1
  [usq] -> Scope2/1, control_AC_voltage1/1(usq)
  Constant2/1 -> control_AC_voltage1/2(usqref)
  Add7/1 -> Scope/1, Gain1/1
  Sum2/1 -> Gain2/1
  Constant3/1 -> Sum2/2
  Gain1/1 -> Sum2/1
  Sum/1 -> control_AC_voltage/2(usdref)
  Constant1/1 -> Sum/1

== system M4B11_modified_AGC_PI/ES4/output ==
  is_xy : Inport
  Pe : Inport  Port=2
  Brecx : Constant  Value=0
  Brecy : Constant  Value=0
  Bus Creator : BusCreator  Inputs=4
  Constant : Constant
  Gain : Gain  Gain=SvscB./SgridB
  Gain1 : Gain  Gain=-1
  Gain2 : Gain  Gain=-1
  Gain6 : Gain
  Grecx : Constant  Value=0
  Grecy : Constant  Value=0
  Mux3 : Mux
  Sum : Sum  Inputs=|++
  m : Outport
  isxy : Outport  Port=2
  GBxy : Outport  Port=3
  wires:
  Bus Creator/1 -> m/1
  Gain6/1 -> GBxy/1, Bus Creator/4  "GBxy"
  Mux3/1 -> Gain6/1
  Grecx/1 -> Mux3/1
  Brecx/1 -> Mux3/3
  Grecy/1 -> Mux3/2
  Brecy/1 -> Mux3/4
  Gain1/1 -> isxy/1, Bus Creator/1  "is_xy"
  Gain2/1 -> Bus Creator/2  "Pe"
  Gain/1 -> Gain1/1  "is_xy"
  Pe/1 -> Gain2/1  "Pe"
  Constant/1 -> Sum/2
  [WreES4] -> Sum/1  "Pe"
  Sum/1 -> Bus Creator/3  "w"
  is_xy/1 -> Gain/1

== system M4B11_modified_AGC_PI/ES4/xy->dq ==
  Ixy : Inport
  Theta : Inport  Port=2
  Complex to Magnitude-Angle : ComplexToMagnitudeAngle
  Complex to Real-Imag : ComplexToRealImag
  Demux1 : Demux  Outputs=2
      settings: DisplayOption=none
  Magnitude-Angle to Complex : MagnitudeAngleToComplex
  Mux : Mux  Inputs=2
  Real-Imag to Complex : RealImagToComplex
  Scope : Scope
      settings: ActiveDisplayYMinimum=3.11918  ActiveDisplayYMaximum=3.16079
  Scope1 : Scope
      settings: ActiveDisplayYMinimum=2.59405  ActiveDisplayYMaximum=3.13201  DataLoggingVariableName=ScopeData3
  Sum1 : Sum  Inputs=|+-  SaturateOnIntegerOverflow=on
  Idq : Outport
  wires:
  Complex to Magnitude-Angle/1 -> Magnitude-Angle to Complex/1
  Theta/1 -> Sum1/2
  Complex to Magnitude-Angle/2 -> Sum1/1, Scope1/1
  Demux1/1 -> Real-Imag to Complex/1
  Complex to Real-Imag/2 -> Mux/2  "Iq"
  Mux/1 -> Idq/1
  Complex to Real-Imag/1 -> Mux/1  "Id"
  Magnitude-Angle to Complex/1 -> Complex to Real-Imag/1
  Sum1/1 -> Magnitude-Angle to Complex/2, Scope/1
  Demux1/2 -> Real-Imag to Complex/2
  Real-Imag to Complex/1 -> Complex to Magnitude-Angle/1
  Ixy/1 -> Demux1/1

== system M4B11_modified_AGC_PI/Generator1/Excitation System ==
  note: Ef
  Upss : Inport
  Trip : Inport  Port=2
  Vg : Inport  Port=3
  Constant : Constant  Value=0
  KA : Gain  Gain=Ka  SaturateOnIntegerOverflow=on  OutDataTypeStr=Inherit: Same as input  ParamDataTypeStr=Inherit: Same as input
  Saturation : Saturate  UpperLimit=Efmax  LowerLimit=Efmin
  Scope : Scope  NumInputPorts=2
      settings: ActiveDisplayYMinimum=0.90537  ActiveDisplayYMaximum=1.09876  DataLoggingVariableName=ScopeData2
  Sum4 : Sum  Inputs=+-+  SaturateOnIntegerOverflow=on
  Switch : Switch  Criteria=u2 ~= 0  Threshold=0.5  InputSameDT=off
  Vref : Constant  Value=Vref
  Ef : Outport
  wires:
  Trip/1 -> Switch/2
  Constant/1 -> Switch/1
  Switch/1 -> Ef/1
  Saturation/1 -> Switch/3
  Sum4/1 -> KA/1
  KA/1 -> Saturation/1
  Vg/1 -> Sum4/2, Scope/2
  Upss/1 -> Sum4/3
  Vref/1 -> Scope/1, Sum4/1

== system M4B11_modified_AGC_PI/Generator1/Governor ==
  w : Inport
  Trip : Inport  Port=2
  CT : Constant  Value=0
  Constant : Constant  Value=0
  Gain1 : Gain  Gain=1/R  SaturateOnIntegerOverflow=on  OutDataTypeStr=Inherit: Same as input  ParamDataTypeStr=Inherit: Same as input
  Saturation : Saturate  UpperLimit=dPmax  LowerLimit=dPmin
  Sum3 : Sum  Inputs=|+-  SaturateOnIntegerOverflow=on
  Switch : Switch  Threshold=0.5  InputSameDT=off
  Switch1 : Switch  Criteria=u2 ~= 0  Threshold=0.5  InputSameDT=off
  Transfer Fcn1 : TransferFcn  Denominator=[Ts_G 1]
  Transfer Fcn2 : TransferFcn  Numerator=[T3_G 1]  Denominator=[Tc_G 1]
  Transfer Fcn3 : TransferFcn  Numerator=[T4_G 1]  Denominator=[T5_G 1]
  w1 : Constant  Value=S_Gov
  wref : Constant
  dPm : Outport
  wires:
  Constant/1 -> Switch1/1
  Switch/1 -> Switch1/3
  Trip/1 -> Switch1/2
  Switch1/1 -> dPm/1
  CT/1 -> Switch/3
  w1/1 -> Switch/2
  wref/1 -> Sum3/1
  w/1 -> Sum3/2
  Saturation/1 -> Switch/1
  Sum3/1 -> Gain1/1
  Gain1/1 -> Transfer Fcn1/1
  Transfer Fcn1/1 -> Transfer Fcn2/1
  Transfer Fcn2/1 -> Transfer Fcn3/1
  Transfer Fcn3/1 -> Saturation/1

== system M4B11_modified_AGC_PI/Generator1/Machine Equations  ==
  note: Idg
  note: Iqg
  delta : Inport
  Vgxy : Inport  Port=2
  Ef : Inport  Port=3
  Trip : Inport  Port=4
  Demux : Demux  Outputs=2
  Demux1 : Demux  Outputs=2
  Fcn1 : Fcn  Expr=u(1)*u(3)+u(2)*u(4)
  Fcn2 : Fcn  Expr=(u(3)-u(2))/Xd11
  Fcn3 : Fcn  Expr=(u(1)-u(4))/Xq11
  Fcn4 : Fcn  Expr=u(2)*u(3)-u(1)*u(4)
  Fcn6 : Fcn  Expr=sqrt(u(1)^2+u(2)^2)
  Interface : Subsystem
  Mux1 : Mux  Inputs=2
  Mux2 : Mux  Inputs=2
  Mux3 : Mux  Inputs=2
  Qe : Scope
      settings: TimeSpan=10  ActiveDisplayYMinimum=-41.36305  ActiveDisplayYMaximum=4.99202
  Scope{,1..3} (4 alike) : Scope
      Scope settings: ActiveDisplayYMinimum=-40.94684  ActiveDisplayYMaximum=4.93423
      Scope1 settings: ActiveDisplayYMinimum=0.69416  ActiveDisplayYMaximum=0.73364  DataLoggingVariableName=ScopeData2
      Scope2 settings: ActiveDisplayYMinimum=0.99148  ActiveDisplayYMaximum=1.03428  DataLoggingVariableName=ScopeData3
      Scope3 settings: ActiveDisplayYMinimum=3.59596  ActiveDisplayYMaximum=3.95434  DataLoggingVariableName=ScopeData4
  Transient Equations : Subsystem
  Pe : Outport
  Igxy1 : Outport  Port=2
  GBxy : Outport  Port=3
  Vg : Outport  Port=4
  wires:
  Fcn3/1 -> Mux3/2
  Fcn2/1 -> Mux3/1
  Mux3/1 -> Demux1/1, Mux2/2, Transient Equations/1(Idqg)
  Interface/1(Vdqg) -> Demux/1, Mux2/1, Fcn6/1, Mux1/1
  Mux1/1 -> Fcn2/1, Fcn3/1
  Mux2/1 -> Fcn1/1, Fcn4/1
  Ef/1 -> Transient Equations/2(Ef)
  Fcn1/1 -> Pe/1
  Fcn6/1 -> Vg/1
  Fcn4/1 -> Qe/1
  delta/1 -> Interface/1(delta)
  Vgxy/1 -> Interface/2(Vgxy)
  Interface/2(Igxy1) -> Igxy1/1
  Interface/3(GBxy) -> GBxy/1
  Transient Equations/1(Eqd'') -> Mux1/2, Interface/3(Eqd'')
  Demux/1 -> Scope1/1
  Demux1/1 -> Scope/1
  Demux/2 -> Scope2/1
  Demux1/2 -> Scope3/1
  Trip/1 -> [Trip]
  [Trip] -> Transient Equations/3(Trip)

== system M4B11_modified_AGC_PI/Generator1/Mechanical DE ==
  Pe : Inport
  dPm : Inport  Port=2
  Trip : Inport  Port=3
  Constant1 : Constant  Value=0
  Constant2 : Constant  Value=0
  Gain : Gain  Gain=wB  SaturateOnIntegerOverflow=on  OutDataTypeStr=Inherit: Same as input  ParamDataTypeStr=Inherit: Same as input
  Gain1 : Gain  Gain=1/H  SaturateOnIntegerOverflow=on  OutDataTypeStr=Inherit: Same as input  ParamDataTypeStr=Inherit: Same as input
  Gain2 : Gain  Gain=D  SaturateOnIntegerOverflow=on  OutDataTypeStr=Inherit: Same as input  ParamDataTypeStr=Inherit: Same as input
  Gain5 : Gain  Gain=180/pi  SaturateOnIntegerOverflow=on  OutDataTypeStr=Inherit: Same as input  ParamDataTypeStr=Inherit: Same as input
  Int1 : Integrator  InitialCondition=delta0
  Int2 : Integrator  InitialCondition=w0
  Pm : Constant  Value=Pm0
  Scope2 : Scope
      settings: TimeSpan=10  ActiveDisplayYMinimum=-0.4  ActiveDisplayYMaximum=1.4  DataLoggingVariableName=ScopeData5
  Scope4 : Scope
      settings: TimeSpan=10  ActiveDisplayYMinimum=0.99397  ActiveDisplayYMaximum=1.02044  DataLoggingVariableName=ScopeData6
  Scope8 : Scope
      settings: TimeSpan=10  ActiveDisplayYMinimum=-0.4  ActiveDisplayYMaximum=1.4  DataLoggingVariableName=ScopeData11
  Sum2 : Sum  Inputs=-+-+  SaturateOnIntegerOverflow=on
  Sum3 : Sum  Inputs=|+-  SaturateOnIntegerOverflow=on
  Switch{1..4} (4 alike) : Switch  Criteria=u2 ~= 0  Threshold=0.5  InputSameDT=off
  w0 : Constant
  delta : Outport
  w : Outport  Port=2
  wires:
  [Trip] -> Switch3/2, Switch2/2
  Constant1/1 -> Switch3/1, Switch2/1
  Switch3/1 -> Scope4/1, Sum3/1, w/1
  Int2/1 -> Switch3/3
  Switch2/1 -> Int2/1
  Gain1/1 -> Switch2/3
  Trip/1 -> [Trip]
  [Trip] -> Switch1/2, Switch4/2
  Constant2/1 -> Switch4/1, Switch1/1
  Switch4/1 -> delta/1, Scope2/1, Gain5/1
  Int1/1 -> Switch4/3
  Switch1/1 -> Int1/1
  Gain/1 -> Switch1/3
  Gain5/1 -> Scope8/1
  w0/1 -> Sum3/2
  Sum3/1 -> Gain2/1, Gain/1
  Pm/1 -> Sum2/2
  Gain2/1 -> Sum2/1
  Sum2/1 -> Gain1/1
  Pe/1 -> Sum2/3
  dPm/1 -> Sum2/4

== system M4B11_modified_AGC_PI/Generator1/Output ==
  Igxy1in : Inport
  GBxyin : Inport  Port=2
  deltain : Inport  Port=3
  Pein : Inport  Port=4
  fin : Inport  Port=5
  Vg : Inport  Port=6
  Bus Creator : BusCreator  Inputs=6
  m : Outport
  Igxy1 : Outport  Port=2
  GBxy : Outport  Port=3
  wires:
  Bus Creator/1 -> m/1
  Igxy1in/1 -> Igxy1/1, Bus Creator/1  "Igxy1"
  GBxyin/1 -> GBxy/1, Bus Creator/2  "GBxy"
  deltain/1 -> Bus Creator/3  "delta"
  Pein/1 -> Bus Creator/4  "Pe"
  fin/1 -> Bus Creator/5  "f"
  Vg/1 -> Bus Creator/6  "Vg"

== system M4B11_modified_AGC_PI/Generator1/PSS1 ==
  w : Inport
  Trip : Inport  Port=2
  CT : Constant  Value=0
  Constant : Constant  Value=0
  Gain : Gain  Gain=Kpss  SaturateOnIntegerOverflow=on  OutDataTypeStr=Inherit: Same as input  ParamDataTypeStr=Inherit: Same as input
  Saturation : Saturate  UpperLimit=Upmax  LowerLimit=Upmin
  Sum3 : Sum  Inputs=|+-  SaturateOnIntegerOverflow=on
  Switch : Switch  Threshold=0.5  InputSameDT=off
  Switch1 : Switch  Threshold=0.5  InputSameDT=off
  Transfer Fcn : TransferFcn  Numerator=[Tw_P 0]  Denominator=[Tw_P 1]
  Transfer Fcn1 : TransferFcn  Numerator=[T1_P 1]  Denominator=[T2_P 1]
  Transfer Fcn2 : TransferFcn  Numerator=[T3_P 1]  Denominator=[T4_P 1]
  w0 : Constant
  w1 : Constant  Value=S_PSS
  Upss : Outport
  wires:
  Constant/1 -> Switch1/1
  Trip/1 -> Switch1/2
  Switch1/1 -> Upss/1
  Switch/1 -> Switch1/3
  Transfer Fcn/1 -> Transfer Fcn1/1
  Gain/1 -> Transfer Fcn/1
  w1/1 -> Switch/2
  CT/1 -> Switch/3
  Saturation/1 -> Switch/1
  Sum3/1 -> Gain/1
  Transfer Fcn2/1 -> Saturation/1
  Transfer Fcn1/1 -> Transfer Fcn2/1
  w/1 -> Sum3/1
  w0/1 -> Sum3/2

== system M4B11_modified_AGC_PI/Generator2/Excitation System ==
  note: Ef
  Upss : Inport
  Trip : Inport  Port=2
  Vg : Inport  Port=3
  Constant : Constant  Value=0
  KA : Gain  Gain=Ka  SaturateOnIntegerOverflow=on  OutDataTypeStr=Inherit: Same as input  ParamDataTypeStr=Inherit: Same as input
  Saturation : Saturate  UpperLimit=Efmax  LowerLimit=Efmin
  Scope : Scope  NumInputPorts=2
      settings: ActiveDisplayYMinimum=0.90537  ActiveDisplayYMaximum=1.09876  DataLoggingVariableName=ScopeData2
  Sum4 : Sum  Inputs=+-+  SaturateOnIntegerOverflow=on
  Switch : Switch  Criteria=u2 ~= 0  Threshold=0.5  InputSameDT=off
  Vref : Constant  Value=Vref
  Ef : Outport
  wires:
  Trip/1 -> Switch/2
  Constant/1 -> Switch/1
  Switch/1 -> Ef/1
  Saturation/1 -> Switch/3
  Sum4/1 -> KA/1
  KA/1 -> Saturation/1
  Vg/1 -> Sum4/2, Scope/2
  Upss/1 -> Sum4/3
  Vref/1 -> Scope/1, Sum4/1

== system M4B11_modified_AGC_PI/Generator2/Governor ==
  w : Inport
  Trip : Inport  Port=2
  CT : Constant  Value=0
  Constant : Constant  Value=0
  Gain1 : Gain  Gain=1/R  SaturateOnIntegerOverflow=on  OutDataTypeStr=Inherit: Same as input  ParamDataTypeStr=Inherit: Same as input
  Saturation : Saturate  UpperLimit=dPmax  LowerLimit=dPmin
  Sum3 : Sum  Inputs=|+-  SaturateOnIntegerOverflow=on
  Switch : Switch  Threshold=0.5  InputSameDT=off
  Switch1 : Switch  Criteria=u2 ~= 0  Threshold=0.5  InputSameDT=off
  Transfer Fcn1 : TransferFcn  Denominator=[Ts_G 1]
  Transfer Fcn2 : TransferFcn  Numerator=[T3_G 1]  Denominator=[Tc_G 1]
  Transfer Fcn3 : TransferFcn  Numerator=[T4_G 1]  Denominator=[T5_G 1]
  w1 : Constant  Value=S_Gov
  wref : Constant
  dPm : Outport
  wires:
  Constant/1 -> Switch1/1
  Switch/1 -> Switch1/3
  Trip/1 -> Switch1/2
  Switch1/1 -> dPm/1
  CT/1 -> Switch/3
  w1/1 -> Switch/2
  wref/1 -> Sum3/1
  w/1 -> Sum3/2
  Saturation/1 -> Switch/1
  Sum3/1 -> Gain1/1
  Gain1/1 -> Transfer Fcn1/1
  Transfer Fcn1/1 -> Transfer Fcn2/1
  Transfer Fcn2/1 -> Transfer Fcn3/1
  Transfer Fcn3/1 -> Saturation/1

== system M4B11_modified_AGC_PI/Generator2/Machine Equations  ==
  note: Idg
  note: Iqg
  delta : Inport
  Vgxy : Inport  Port=2
  Ef : Inport  Port=3
  Trip : Inport  Port=4
  Demux : Demux  Outputs=2
  Demux1 : Demux  Outputs=2
  Fcn1 : Fcn  Expr=u(1)*u(3)+u(2)*u(4)
  Fcn2 : Fcn  Expr=(u(3)-u(2))/Xd11
  Fcn3 : Fcn  Expr=(u(1)-u(4))/Xq11
  Fcn4 : Fcn  Expr=u(2)*u(3)-u(1)*u(4)
  Fcn6 : Fcn  Expr=sqrt(u(1)^2+u(2)^2)
  Interface : Subsystem
  Mux1 : Mux  Inputs=2
  Mux2 : Mux  Inputs=2
  Mux3 : Mux  Inputs=2
  Qe : Scope
      settings: TimeSpan=10  ActiveDisplayYMinimum=-41.36305  ActiveDisplayYMaximum=4.99202
  Scope{,1..3} (4 alike) : Scope
      Scope settings: ActiveDisplayYMinimum=-40.94684  ActiveDisplayYMaximum=4.93423
      Scope1 settings: ActiveDisplayYMinimum=-0.02752  ActiveDisplayYMaximum=0.14126  DataLoggingVariableName=ScopeData2
      Scope2 settings: ActiveDisplayYMinimum=0.99148  ActiveDisplayYMaximum=1.03428  DataLoggingVariableName=ScopeData3
      Scope3 settings: ActiveDisplayYMinimum=3.59596  ActiveDisplayYMaximum=3.95434  DataLoggingVariableName=ScopeData4
  Transient Equations : Subsystem
  Pe : Outport
  Igxy1 : Outport  Port=2
  GBxy : Outport  Port=3
  Vg : Outport  Port=4
  wires:
  Fcn3/1 -> Mux3/2
  Fcn2/1 -> Mux3/1
  Mux3/1 -> Demux1/1, Mux2/2, Transient Equations/1(Idqg)
  Interface/1(Vdqg) -> Demux/1, Mux2/1, Fcn6/1, Mux1/1
  Mux1/1 -> Fcn2/1, Fcn3/1
  Mux2/1 -> Fcn1/1, Fcn4/1
  Ef/1 -> Transient Equations/2(Ef)
  Fcn1/1 -> Pe/1
  Fcn6/1 -> Vg/1
  Fcn4/1 -> Qe/1
  delta/1 -> Interface/1(delta)
  Vgxy/1 -> Interface/2(Vgxy)
  Interface/2(Igxy1) -> Igxy1/1
  Interface/3(GBxy) -> GBxy/1
  Transient Equations/1(Eqd'') -> Mux1/2, Interface/3(Eqd'')
  Demux/1 -> Scope1/1
  Demux1/1 -> Scope/1
  Demux/2 -> Scope2/1
  Demux1/2 -> Scope3/1
  Trip/1 -> [Trip]
  [Trip] -> Transient Equations/3(Trip)

== system M4B11_modified_AGC_PI/Generator2/Mechanical DE ==
  Pe : Inport
  dPm : Inport  Port=2
  Trip : Inport  Port=3
  Constant1 : Constant  Value=0
  Constant2 : Constant  Value=0
  Gain : Gain  Gain=wB  SaturateOnIntegerOverflow=on  OutDataTypeStr=Inherit: Same as input  ParamDataTypeStr=Inherit: Same as input
  Gain1 : Gain  Gain=1/H  SaturateOnIntegerOverflow=on  OutDataTypeStr=Inherit: Same as input  ParamDataTypeStr=Inherit: Same as input
  Gain2 : Gain  Gain=D  SaturateOnIntegerOverflow=on  OutDataTypeStr=Inherit: Same as input  ParamDataTypeStr=Inherit: Same as input
  Gain5 : Gain  Gain=180/pi  SaturateOnIntegerOverflow=on  OutDataTypeStr=Inherit: Same as input  ParamDataTypeStr=Inherit: Same as input
  Int1 : Integrator  InitialCondition=delta0
  Int2 : Integrator  InitialCondition=w0
  Pm : Constant  Value=Pm0
  Scope2 : Scope
      settings: TimeSpan=10  ActiveDisplayYMinimum=-0.4  ActiveDisplayYMaximum=1.4  DataLoggingVariableName=ScopeData5
  Scope4 : Scope
      settings: TimeSpan=10  ActiveDisplayYMinimum=0.99397  ActiveDisplayYMaximum=1.02044  DataLoggingVariableName=ScopeData6
  Scope8 : Scope
      settings: TimeSpan=10  ActiveDisplayYMinimum=-0.4  ActiveDisplayYMaximum=1.4  DataLoggingVariableName=ScopeData11
  Sum2 : Sum  Inputs=-+-+  SaturateOnIntegerOverflow=on
  Sum3 : Sum  Inputs=|+-  SaturateOnIntegerOverflow=on
  Switch{1..4} (4 alike) : Switch  Criteria=u2 ~= 0  Threshold=0.5  InputSameDT=off
  w0 : Constant
  delta : Outport
  w : Outport  Port=2
  wires:
  [Trip] -> Switch3/2, Switch2/2
  Constant1/1 -> Switch3/1, Switch2/1
  Switch3/1 -> Scope4/1, Sum3/1, w/1
  Int2/1 -> Switch3/3
  Switch2/1 -> Int2/1
  Gain1/1 -> Switch2/3
  Trip/1 -> [Trip]
  [Trip] -> Switch1/2, Switch4/2
  Constant2/1 -> Switch4/1, Switch1/1
  Switch4/1 -> delta/1, Scope2/1, Gain5/1
  Int1/1 -> Switch4/3
  Switch1/1 -> Int1/1
  Gain/1 -> Switch1/3
  Gain5/1 -> Scope8/1
  w0/1 -> Sum3/2
  Sum3/1 -> Gain2/1, Gain/1
  Pm/1 -> Sum2/2
  Gain2/1 -> Sum2/1
  Sum2/1 -> Gain1/1
  Pe/1 -> Sum2/3
  dPm/1 -> Sum2/4

== system M4B11_modified_AGC_PI/Generator2/Output ==
  Igxy1in : Inport
  GBxyin : Inport  Port=2
  deltain : Inport  Port=3
  Pein : Inport  Port=4
  fin : Inport  Port=5
  Vg : Inport  Port=6
  Bus Creator : BusCreator  Inputs=6
  m : Outport
  Igxy1 : Outport  Port=2
  GBxy : Outport  Port=3
  wires:
  Bus Creator/1 -> m/1
  Igxy1in/1 -> Igxy1/1, Bus Creator/1  "Igxy1"
  GBxyin/1 -> GBxy/1, Bus Creator/2  "GBxy"
  deltain/1 -> Bus Creator/3  "delta"
  Pein/1 -> Bus Creator/4  "Pe"
  fin/1 -> Bus Creator/5  "f"
  Vg/1 -> Bus Creator/6  "Vg"

== system M4B11_modified_AGC_PI/Generator2/PSS1 ==
  w : Inport
  Trip : Inport  Port=2
  CT : Constant  Value=0
  Constant : Constant  Value=0
  Gain : Gain  Gain=Kpss  SaturateOnIntegerOverflow=on  OutDataTypeStr=Inherit: Same as input  ParamDataTypeStr=Inherit: Same as input
  Saturation : Saturate  UpperLimit=Upmax  LowerLimit=Upmin
  Sum3 : Sum  Inputs=|+-  SaturateOnIntegerOverflow=on
  Switch : Switch  Threshold=0.5  InputSameDT=off
  Switch1 : Switch  Threshold=0.5  InputSameDT=off
  Transfer Fcn : TransferFcn  Numerator=[Tw_P 0]  Denominator=[Tw_P 1]
  Transfer Fcn1 : TransferFcn  Numerator=[T1_P 1]  Denominator=[T2_P 1]
  Transfer Fcn2 : TransferFcn  Numerator=[T3_P 1]  Denominator=[T4_P 1]
  w0 : Constant
  w1 : Constant  Value=S_PSS
  Upss : Outport
  wires:
  Constant/1 -> Switch1/1
  Trip/1 -> Switch1/2
  Switch1/1 -> Upss/1
  Switch/1 -> Switch1/3
  Transfer Fcn/1 -> Transfer Fcn1/1
  Gain/1 -> Transfer Fcn/1
  w1/1 -> Switch/2
  CT/1 -> Switch/3
  Saturation/1 -> Switch/1
  Sum3/1 -> Gain/1
  Transfer Fcn2/1 -> Saturation/1
  Transfer Fcn1/1 -> Transfer Fcn2/1
  w/1 -> Sum3/1
  w0/1 -> Sum3/2
